simulink model "Project2ss_not_used"  (R2019a)
settings: Solver=VariableStepAuto  StartTime=0.0  StopTime=10.0  RelTol=1e-3
undefined symbols (not defined in the file): au_C, DiscIntNeverNeededParam, Discrete, dt, filter_R, plant_A, plant_B, plant_C, plant_D, sensor_tf, sf_gains, Time
libraries: ctrlSharedLib x1
settings Model: Creator=crs20  LastModifiedBy=crs20

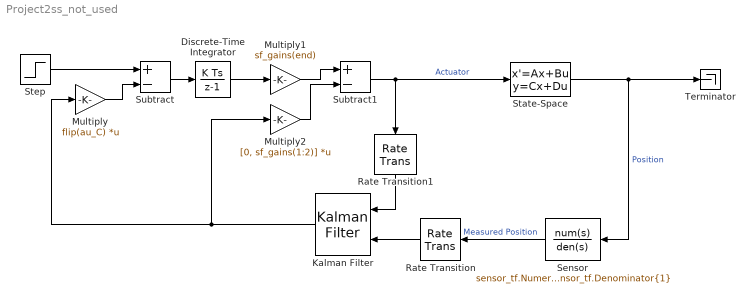
== system Project2ss_not_used ==
  Discrete-Time Integrator : DiscreteIntegrator  SampleTime=dt  ICPrevOutput=DiscIntNeverNeededParam  ICPrevScaledInput=DiscIntNeverNeededParam
  Kalman Filter : ctrlSharedLib/Kalman Filter  TimeDomain=Discrete-Time  UseCurrentEstimator=on  ModelSource=LTI State-Space Variable  ModelSourceVariable=filter_ss  A=0.95  B=1  C=1  D=0  NumberOfStates=1  NumberOfInputs=1  NumberOfOutputs=1  InitialEstimateSource=Dialog  X0=0  P0=10  UseK=off  UseGH=off  NumberOfProcessNoiseInputs=1  G=1  TimeInvariantG=on  H=0  TimeInvariantH=on  Q=filter_Q  TimeInvariantQ=on  R=filter_R  TimeInvariantR=on  N=0  TimeInvariantN=on  AddInputPort=on  AddEnablePort=off  OutputEstimatedY=off  OutputP=off  Ts=-1
      settings: SourceProductBaseCode=CT
  Multiply : Gain  Gain=flip(au_C)  Multiplication=Matrix(K*u)
  Multiply1 : Gain  Gain=sf_gains(end)
  Multiply2 : Gain  Gain=[0, sf_gains(1:2)]  Multiplication=Matrix(K*u)
  Rate Transition : RateTransition
  Rate Transition1 : RateTransition
  Sensor : TransferFcn  Numerator=sensor_tf.Numerator{1}  Denominator=sensor_tf.Denominator{1}
  State-Space : StateSpace  A=plant_A  B=plant_B  C=plant_C  D=plant_D  InitialCondition=0
  Step : Step  Time=0  SampleTime=0
  Subtract : Sum  Inputs=+-
  Subtract1 : Sum  Inputs=+-
  Terminator : Terminator
  wires:
  State-Space/1 -> Terminator/1, Sensor/1  "Position"
  Sensor/1 -> Rate Transition/1  "Measured Position"
  Rate Transition/1 -> Kalman Filter/2
  Rate Transition1/1 -> Kalman Filter/1
  Step/1 -> Subtract/1
  Kalman Filter/1 -> Multiply2/1, Multiply/1
  Subtract1/1 -> State-Space/1, Rate Transition1/1  "Actuator"
  Multiply/1 -> Subtract/2
  Discrete-Time Integrator/1 -> Multiply1/1
  Subtract/1 -> Discrete-Time Integrator/1
  Multiply1/1 -> Subtract1/1
  Multiply2/1 -> Subtract1/2
